simulink model "st_re"  (R2017b)
settings: Solver=VariableStepAuto  StartTime=0.0  StopTime=10  MaxStep=1e-4  RelTol=1e-3
settings Model: Creator=Administrator  LastModifiedBy=Administrator

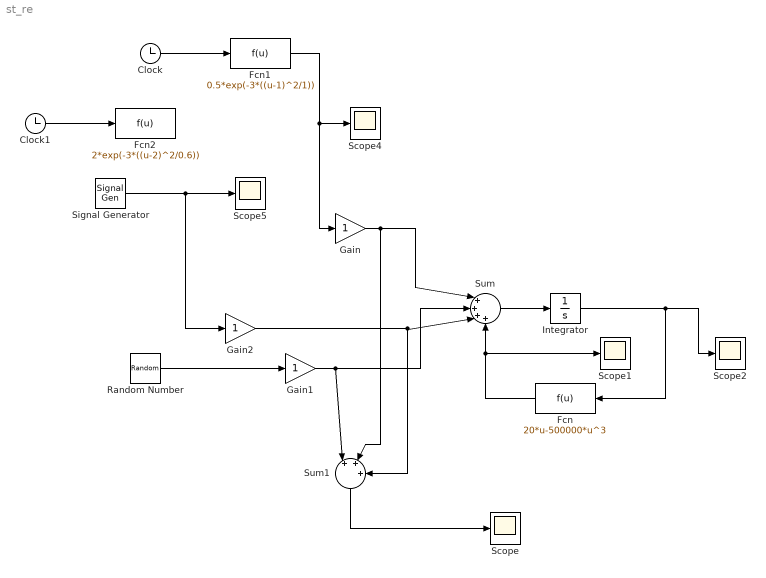
== system st_re ==
  Clock : Clock
  Clock1 : Clock
  Fcn : Fcn  Expr=20*u-500000*u^3
  Fcn1 : Fcn  Expr=0.5*exp(-3*((u-1)^2/1))
  Fcn2 : Fcn  Expr=2*exp(-3*((u-2)^2/0.6))
  Gain : Gain
  Gain1 : Gain
  Gain2 : Gain
  Integrator : Integrator
  Random Number : RandomNumber  Variance=2  SampleTime=0.0
  Scope{,1..2,4..5} (5 alike) : Scope
  Signal Generator : SignalGenerator  Amplitude=0.4  Frequency=20  Units=rad/sec
  Sum : Sum  Inputs=|++++
  Sum1 : Sum  Inputs=|+++
  wires:
  Gain1/1 -> Sum1/1, Sum/2
  Gain/1 -> Sum1/2, Sum/1
  Fcn/1 -> Sum/4, Scope1/1
  Sum/1 -> Integrator/1
  Integrator/1 -> Scope2/1, Fcn/1
  Sum1/1 -> Scope/1
  Random Number/1 -> Gain1/1
  Clock/1 -> Fcn1/1
  Fcn1/1 -> Gain/1, Scope4/1
  Clock1/1 -> Fcn2/1
  Gain2/1 -> Sum1/3, Sum/3
  Signal Generator/1 -> Gain2/1, Scope5/1
